simulink library "ControLibrary"  (R2015b)
settings: Solver=ode45  SolverMode=SingleTasking  StartTime=0.0  StopTime=10.0  RelTol=1e-3
values from neighbouring files (symbols this model uses):
  ControlSampleTime = 1/8000    (= 0.000125)    [initTPHardware.m]
  DCCC = initDCCC(LCL,SM)    [Sim_TP3_VSM_init.m]    (also in initDCCC.m = initHSS(LCL,SM))
undefined symbols (not defined in the file or in its folder): CCCTRL, DiscIntNeverNeededParam, VSMCTRL
undefined symbols (not defined in the file): HSS, VSMCC
libraries: FriedrichLibrary x46, simulink x23, simulink_extras x4, ControLibrary x2, ctrl_basic x2
(part 4 of 4)

== system ControLibrary/VSM/CONTROL/VSMOC/VSMOC/Integrator (Inertia) ==
  dPTa : Inport
  omega0 [pu] : Inport  Port=2
  Enable : EnablePort
  Integrator (inertia) : DiscreteIntegrator  gainval=1  InitialConditionSource=external  InitialCondition=1  InitialConditionSetting=State (most efficient)  SampleTime=ControlSampleTime  ICPrevOutput=DiscIntNeverNeededParam  ICPrevScaledInput=DiscIntNeverNeededParam
  omega [pu] : Outport
  wires:
  dPTa/1 -> Integrator (inertia)/1
  Integrator (inertia)/1 -> omega [pu]/1  "Omega [pu]"
  omega0 [pu]/1 -> Integrator (inertia)/2

== system ControLibrary/VSM/CONTROL/VSMOC/VSMOC/P Filter Init ==
  Tau : Inport
  dP0 : Inport  Port=2
  Enable : EnablePort  StatesWhenEnabling=reset
  Divide4 : Product  Inputs=*/
  Gain : Gain  Gain=-1
  Integrator1 : DiscreteIntegrator  gainval=1  InitialConditionSource=external  InitialConditionSetting=State (most efficient)  SampleTime=ControlSampleTime  ICPrevOutput=DiscIntNeverNeededParam  ICPrevScaledInput=DiscIntNeverNeededParam
  dP : Outport
  wires:
  Integrator1/1 -> Gain/1, dP/1
  Tau/1 -> Divide4/2
  Divide4/1 -> Integrator1/1
  Gain/1 -> Divide4/1
  dP0/1 -> Integrator1/2

== system ControLibrary/VSM/CONTROL/VSMOC/VSMOC/Subsystem ==
  first_run : Inport
  u_dq : Inport  Port=2
  u_dq_pll : Inport  Port=3
  phi_pll : Inport  Port=4
  Enable : EnablePort
  Complex to Magnitude-Angle : ComplexToMagnitudeAngle
  Demux : Demux  Outputs=2
  Real-Imag to Complex : RealImagToComplex
  Switch : Switch  Criteria=u2 > Threshold
  Switch1 : Switch  Criteria=u2 ~= 0
  "first_run " : InportShadow
  u_abs : Outport  InitialOutput=1
  u_ang : Outport  Port=2  InitialOutput=0
  wires:
  Complex to Magnitude-Angle/2 -> Switch/3
  "first_run "/1 -> Switch/2
  u_dq_pll/1 -> Switch1/1
  u_dq/1 -> Switch1/3
  first_run/1 -> Switch1/2
  Switch1/1 -> Demux/1
  Complex to Magnitude-Angle/1 -> u_abs/1
  Demux/2 -> Real-Imag to Complex/2
  Demux/1 -> Real-Imag to Complex/1
  Real-Imag to Complex/1 -> Complex to Magnitude-Angle/1
  phi_pll/1 -> Switch/1
  Switch/1 -> u_ang/1

== system ControLibrary/VSM/CONTROL/VSMOC/VSMOC/Tiefpass Statik ==
  1/Tau : Inport
  E : Inport  Port=2
  E0 : Inport  Port=3
  Enable : EnablePort  StatesWhenEnabling=reset
  Divide1 : Product  Inputs=**
  Integrator : DiscreteIntegrator  gainval=1  InitialConditionSource=external  InitialCondition=0.9  InitialConditionSetting=State (most efficient)  SampleTime=ControlSampleTime  ICPrevOutput=DiscIntNeverNeededParam  ICPrevScaledInput=DiscIntNeverNeededParam
  Sum6 : Sum  Inputs=|+-
  E_fil : Outport
  wires:
  1/Tau/1 -> Divide1/1
  Sum6/1 -> Divide1/2
  Divide1/1 -> Integrator/1
  E/1 -> Sum6/1
  Integrator/1 -> Sum6/2, E_fil/1  "E [pu]"
  E0/1 -> Integrator/2

== system ControLibrary/VSM/MANAGEMENT/sp_VSM/RateLimit/ratelimitspPQ ==
  rateup : Inport
  x : Inport  Port=2
  ratedown : Inport  Port=3
  x0 : Inport  Port=4
  Delay : Delay  DelayLength=1  InitialConditionSource=Input port  SampleTime=Ts
      settings: InputPortMap=u0,p4
  Gain : Gain  Gain=Ts
  Gain1 : Gain  Gain=-Ts
  Saturation Dynamic2 : simulink/Discontinuities/Saturation Dynamic  OutMin=[]  OutMax=[]  OutDataTypeStr=Inherit: Same as second input  OutDataType=fixdt(1, 16)  OutScaling=2^-10  DoSatur=off
  Sum : Sum  Inputs=|+-
  Sum1 : Sum  Inputs=|++
  x_slow : Outport
  wires:
  x/1 -> Sum/1
  Delay/1 -> Sum1/2, Sum/2
  Sum/1 -> Saturation Dynamic2/2
  Saturation Dynamic2/1 -> Sum1/1
  Sum1/1 -> x_slow/1, Delay/1
  x0/1 -> Delay/2
  Gain/1 -> Saturation Dynamic2/1
  rateup/1 -> Gain/1
  ratedown/1 -> Gain1/1
  Gain1/1 -> Saturation Dynamic2/3

== matlab function ControLibrary/VSM/CONTROL/re_init/MATLAB Function ==
  data: Uset input; Uinit output; Phi output; Uvr input; UvrShift output
function [Uinit, Phi, UvrShift] = initAngle(Uset,Uvr)
EPSPHI   = 0.1*2*pi/360;
Phi      = 0;
UvrShift = Uvr;

for ICount = 1:10
    Uinit   = Uset + UvrShift;
    PhiOld  = Phi;
    Phi     = atan2(Uinit(2),Uinit(1));
    
    
    if abs(Phi-PhiOld) < EPSPHI
        break
    end
    
    UvrShift(1) = + cos(Phi)*Uvr(1) + sin(Phi)*Uvr(2);
    UvrShift(2) = - sin(Phi)*Uvr(1) + cos(Phi)*Uvr(2);
end
end
